simulink model "Excavator_Mevea_Bucket"  (R2026a)
settings: Solver=ode23t  StopTime=stopTime  FixedStep=1e-5  MaxStep=Ts  AbsTol=1e-3
PostLoadFcn:
  | set_param(bdroot,'IgnoredZcDiagnostic','none');
  | Excavator_Test_Scenario_Select('loadedBucketDigCycle');
  | Excavator_Mevea_params
StartFcn:
  | tStart = tic;
StopFcn:
  | elapsedSimTime = toc(tStart);
  | disp(['Elapsed Sim Time = ' num2str(elapsedSimTime)]);
model workspace: external: MAT-File ExcavatorAssemblyDataStruct.mat (data not in the file)
undefined symbols (not defined in the file or in its folder): AToBRegOrificeVector, AToTOrificeVector, BiPOrificeVector, BoomC, boomHEArea, boomREArea, boomUpMaxQ, boomValve, BToTOrificeVector, BucketC, bucketCloseMaxQ, bucketOpenMaxQ, BucketR, bucketValve, fluids, gravity, LeftBoomR, maxPumpDisp, minPumpDisp, nominalEngineSpeed, P28Assembly, PToAOrificeVector, PToBOrificeVector, pumpCmdNegRateLimit, pumpCmdPosRateLimit, RightBoomR, StickC, stickInMaxQ, stickOutMaxQ, StickR, stickValve, SwingC, swingDisplacement, swingHighSpeedThreshold, swingMaxQ, SwingR, swingSpeedQGain, swingValve, valveCmdNegRateLimit, valveCmdPosRateLimit, X, Y, Z
libraries: fl_lib x89, sm_lib x79, SimscapeFluids_lib x78, nesl_utility x57, simulink_extras x11, Excavator_Parts_Lib x6, SignalEditorBlockLib x1
(part 4 of 7)

== system Excavator_Mevea_Bucket/Excavator/Hydraulics/Functions/Bucket ==
  note: This leakage can be included if necessary.
      | Scale carefully to avoid drift due to gravity.
  BucketCylinder : SimscapeFluids_lib/Isothermal Liquid/Actuators/Double-Acting Actuator (IL)  single_fluid=true  mech_orientation=foundation.enum.MechOrientationTranslational.Positive  piston_area_A=bucketHEArea mm^2  piston_area_B=bucketREArea mm^2  stroke=bucketStroke mm  dead_volume_A=5e-4 m^3  dead_volume_B=5e-4 m^3  pressure_spec=foundation.enum.pressure_spec.atmospheric  environment_pressure=0.101325 MPa  hardstop_model=simscape.enum.hardstop.smooth  stiff_coeff=1e8 N/m  damping_coeff=1e6 N/(m/s)  transition=0.1 mm  coeff_rest=0.7  v_tol=0.001 m/s  f_tol=0.001 N  cushion_A_spec=simscape.enum.onoff.off  area_plunger_A=1e-4 m^2  length_plunger_A=1e-3 m  area_cushion_orifice_A=1e-6 m^2  area_leak_plunger_A=1e-7 m^2  p_crack_differential_A=0.01 MPa  press_max_differential_A=0.1 MPa  check_valve_area_max_A=1e-4 m^2  check_valve_area_leak_A=1e-10 m^2  smoothing_factor_A=0  cushion_B_spec=simscape.enum.onoff.off  area_plunger_B=1e-4 m^2  length_plunger_B=1e-3 m  area_cushion_orifice_B=1e-6 m^2  area_leak_plunger_B=1e-7 m^2  p_crack_differential_B=0.01 MPa  press_max_differential_B=0.1 MPa  check_valve_area_max_B=1e-4 m^2  check_valve_area_leak_B=1e-10 m^2  smoothing_factor_B=0  friction_spec=true  breakaway_Coulomb_ratio=bucketCylFriction.brkawyToCoulRatio  breakaway_velocity=bucketCylFriction.brkawyVel m/s  preload_force=bucketCylFriction.preloadForce N  Coulomb_coeff=bucketCylFriction.coulForceCoef N/Pa  viscous_coeff=bucketCylFriction.viscCoeff N/(m/s)  leakage_spec=simscape.enum.onoff.off  clearance=1e-4 m  piston_length=0.01 m  displacement_spec=foundation.enum.DisplacementSpec.Calculate  x0=initBucketPistonPos mm  dynamic_compressibility=simscape.enum.onoff.on  p0_A=initBucketHEPr bar  p0_B=initBucketREPr bar  p_nominal_A=0.101325 MPa  p_nominal_B=0.101325 MPa
  BucketHEPrSensor : fl_lib/Isothermal Liquid/Sensors/Pressure Sensor (IL)  pressure_measure=foundation.enum.pressure_measure.gauge
  BucketREPrSensor : fl_lib/Isothermal Liquid/Sensors/Pressure Sensor (IL)  pressure_measure=foundation.enum.pressure_measure.gauge
  BucketScope : Scope  NumInputPorts=3
      settings: ActiveDisplayYMinimum=-87.77863  ActiveDisplayYMaximum=1124.28313  DataLoggingVariableName=ScopeData2
  BucketTranslationalRef : fl_lib/Mechanical/Translational Elements/Mechanical Translational Reference
  Laminar Leakage (IL)1 : fl_lib/Isothermal Liquid/Elements/Laminar Leakage (IL)  Commented=on  cross_section_geometry=foundation.enum.cross_section_geometry.annular  diameter=1e-3 m  inner_diameter=bucketBoreDiameter-pistonCylClearance mm  outer_diameter=bucketBoreDiameter mm  width=1e-3 m  height=0.1 m  major_axis=1e-3 m  minor_axis=5e-4 m  side_length=1e-3 m  length=pistonHeadLen mm  resistance=1e3 MPa*s/m^3
  PS-Simulink Converter : nesl_utility/PS-Simulink Converter  PhysicalDomain=network_engine_domain  SubClassName=ps_output  LeftPortType=input  RightPortType=output  PseudoPeriodic=off  Frequencies=[]  VectorFormat=1-D array  Unit=bar  AffineConversion=off
  PS-Simulink Converter1 : nesl_utility/PS-Simulink Converter  PhysicalDomain=network_engine_domain  SubClassName=ps_output  LeftPortType=input  RightPortType=output  PseudoPeriodic=off  Frequencies=[]  VectorFormat=1-D array  Unit=bar  AffineConversion=off
  PS-Simulink Converter2 : nesl_utility/PS-Simulink Converter  PhysicalDomain=network_engine_domain  SubClassName=ps_output  LeftPortType=input  RightPortType=output  PseudoPeriodic=off  Frequencies=[]  VectorFormat=1-D array  Unit=mm  AffineConversion=off
  Simscape Bus : SimscapeBus  HierarchyStrings=BucketC;BucketR
  Transfer Fcn (with initial outputs) : simulink_extras/Additional Linear/Transfer Fcn (with initial outputs)  N=[1]  D="[0.01  1]"  Y0=initBucketHEPr  U0=initBucketHEPr
  Transfer Fcn (with initial outputs)1 : simulink_extras/Additional Linear/Transfer Fcn (with initial outputs)  N=[1]  D="[0.01  1]"  Y0=initBucketREPr  U0=initBucketREPr
  BucketA : PMIOPort  Side=Left
  BucketB : PMIOPort  Port=2  Side=Left
  BucketHydToMech : PMIOPort  Port=3  Side=Right
  BucketHEPr : Outport
  BucketREPr : Outport  Port=2
  BucketPos : Outport  Port=3
  wires:
  PS-Simulink Converter1/1 -> Transfer Fcn (with initial outputs)/1  "BucketHEPr"
  PS-Simulink Converter/1 -> Transfer Fcn (with initial outputs)1/1  "BucketREPr"
  Transfer Fcn (with initial outputs)/1 -> BucketScope/3, BucketHEPr/1  "BucketHEPr"
  Transfer Fcn (with initial outputs)1/1 -> BucketREPr/1, BucketScope/2  "BucketREPr"
  PS-Simulink Converter2/1 -> BucketScope/1, BucketPos/1  "BucketPos"
  connections:
  Simscape Bus/LConn2 -- BucketCylinder/RConn2
  BucketCylinder/LConn2 -- BucketA/RConn1 -- Laminar Leakage (IL)1/LConn1 -- BucketHEPrSensor/LConn1
  BucketCylinder/LConn1 -- Simscape Bus/LConn1 -- BucketTranslationalRef/LConn1
  BucketREPrSensor/LConn1 -- Laminar Leakage (IL)1/RConn1 -- BucketCylinder/RConn3 -- BucketB/RConn1
  Simscape Bus/RConn1 -- BucketHydToMech/RConn1
  BucketREPrSensor/RConn1 -- PS-Simulink Converter/LConn1
  BucketHEPrSensor/RConn1 -- PS-Simulink Converter1/LConn1
  PS-Simulink Converter2/LConn1 -- BucketCylinder/RConn1

== system Excavator_Mevea_Bucket/Excavator/Hydraulics/Functions/Stick ==
  note: This leakage can be included if necessary.
      | Scale carefully to avoid drift due to gravity.
  Laminar Leakage (IL)1 : fl_lib/Isothermal Liquid/Elements/Laminar Leakage (IL)  Commented=on  cross_section_geometry=foundation.enum.cross_section_geometry.annular  diameter=1e-3 m  inner_diameter=stickBoreDiameter-pistonCylClearance mm  outer_diameter=stickBoreDiameter mm  width=1e-3 m  height=0.1 m  major_axis=1e-3 m  minor_axis=5e-4 m  side_length=1e-3 m  length=pistonHeadLen mm  resistance=1e3 MPa*s/m^3
  PS-Simulink Converter : nesl_utility/PS-Simulink Converter  PhysicalDomain=network_engine_domain  SubClassName=ps_output  LeftPortType=input  RightPortType=output  PseudoPeriodic=off  Frequencies=[]  VectorFormat=1-D array  Unit=bar  AffineConversion=off
  PS-Simulink Converter1 : nesl_utility/PS-Simulink Converter  PhysicalDomain=network_engine_domain  SubClassName=ps_output  LeftPortType=input  RightPortType=output  PseudoPeriodic=off  Frequencies=[]  VectorFormat=1-D array  Unit=bar  AffineConversion=off
  PS-Simulink Converter2 : nesl_utility/PS-Simulink Converter  PhysicalDomain=network_engine_domain  SubClassName=ps_output  LeftPortType=input  RightPortType=output  PseudoPeriodic=off  Frequencies=[]  VectorFormat=1-D array  Unit=mm  AffineConversion=off
  Simscape Bus : SimscapeBus  HierarchyStrings=StickC;StickR
  StickCylinder : SimscapeFluids_lib/Isothermal Liquid/Actuators/Double-Acting Actuator (IL)  single_fluid=true  mech_orientation=foundation.enum.MechOrientationTranslational.Positive  piston_area_A=stickHEArea mm^2  piston_area_B=stickREArea mm^2  stroke=stickStroke mm  dead_volume_A=1e-3 m^3  dead_volume_B=1e-3 m^3  pressure_spec=foundation.enum.pressure_spec.atmospheric  environment_pressure=0.101325 MPa  hardstop_model=simscape.enum.hardstop.smooth  stiff_coeff=1e8 N/m  damping_coeff=1e5 N/(m/s)  transition=0.1 mm  coeff_rest=0.7  v_tol=0.001 m/s  f_tol=0.001 N  cushion_A_spec=simscape.enum.onoff.off  area_plunger_A=1e-4 m^2  length_plunger_A=1e-3 m  area_cushion_orifice_A=1e-6 m^2  area_leak_plunger_A=1e-7 m^2  p_crack_differential_A=0.01 MPa  press_max_differential_A=0.1 MPa  check_valve_area_max_A=1e-4 m^2  check_valve_area_leak_A=1e-10 m^2  smoothing_factor_A=0  cushion_B_spec=simscape.enum.onoff.off  area_plunger_B=1e-4 m^2  length_plunger_B=1e-3 m  area_cushion_orifice_B=1e-6 m^2  area_leak_plunger_B=1e-7 m^2  p_crack_differential_B=0.01 MPa  press_max_differential_B=0.1 MPa  check_valve_area_max_B=1e-4 m^2  check_valve_area_leak_B=1e-10 m^2  smoothing_factor_B=0  friction_spec=simscape.enum.onoff.on  breakaway_Coulomb_ratio=stickCylFriction.brkawyToCoulRatio  breakaway_velocity=stickCylFriction.brkawyVel m/s  preload_force=stickCylFriction.preloadForce N  Coulomb_coeff=stickCylFriction.coulForceCoef N/Pa  viscous_coeff=stickCylFriction.viscCoeff N/(m/s)  leakage_spec=simscape.enum.onoff.off  clearance=1e-4 m  piston_length=0.01 m  displacement_spec=foundation.enum.DisplacementSpec.Calculate  x0=initStickPistonPos mm  dynamic_compressibility=simscape.enum.onoff.on  p0_A=initStickHEPr bar  p0_B=initStickREPr bar  p_nominal_A=0.101325 MPa  p_nominal_B=0.101325 MPa
  StickHEPrSensor : fl_lib/Isothermal Liquid/Sensors/Pressure Sensor (IL)  pressure_measure=foundation.enum.pressure_measure.gauge
  StickREPrSensor : fl_lib/Isothermal Liquid/Sensors/Pressure Sensor (IL)  pressure_measure=foundation.enum.pressure_measure.gauge
  StickTranslationalRef : fl_lib/Mechanical/Translational Elements/Mechanical Translational Reference
  Transfer Fcn (with initial outputs) : simulink_extras/Additional Linear/Transfer Fcn (with initial outputs)  N=[1]  D="[0.01  1]"  Y0=initStickREPr  U0=initStickREPr
  Transfer Fcn (with initial outputs)1 : simulink_extras/Additional Linear/Transfer Fcn (with initial outputs)  N=[1]  D="[0.01  1]"  Y0=initStickHEPr  U0=initStickHEPr
  StickA : PMIOPort  Side=Left
  StickB : PMIOPort  Port=2  Side=Left
  StickHydToMech : PMIOPort  Port=3  Side=Right
  StickHEPr : Outport
  StickREPr : Outport  Port=2
  StickPos : Outport  Port=3
  wires:
  PS-Simulink Converter/1 -> Transfer Fcn (with initial outputs)/1  "StickREPr"
  PS-Simulink Converter1/1 -> Transfer Fcn (with initial outputs)1/1  "StickHEPr"
  Transfer Fcn (with initial outputs)/1 -> StickREPr/1  "StickREPr"
  PS-Simulink Converter2/1 -> StickPos/1  "StickPos"
  Transfer Fcn (with initial outputs)1/1 -> StickHEPr/1  "StickHEPr"
  connections:
  StickCylinder/RConn2 -- Simscape Bus/LConn2
  StickCylinder/RConn3 -- Laminar Leakage (IL)1/RConn1 -- StickREPrSensor/LConn1 -- StickB/RConn1
  StickHEPrSensor/LConn1 -- Laminar Leakage (IL)1/LConn1 -- StickCylinder/LConn2 -- StickA/RConn1
  StickTranslationalRef/LConn1 -- Simscape Bus/LConn1 -- StickCylinder/LConn1
  Simscape Bus/RConn1 -- StickHydToMech/RConn1
  StickREPrSensor/RConn1 -- PS-Simulink Converter/LConn1
  StickHEPrSensor/RConn1 -- PS-Simulink Converter1/LConn1
  PS-Simulink Converter2/LConn1 -- StickCylinder/RConn1

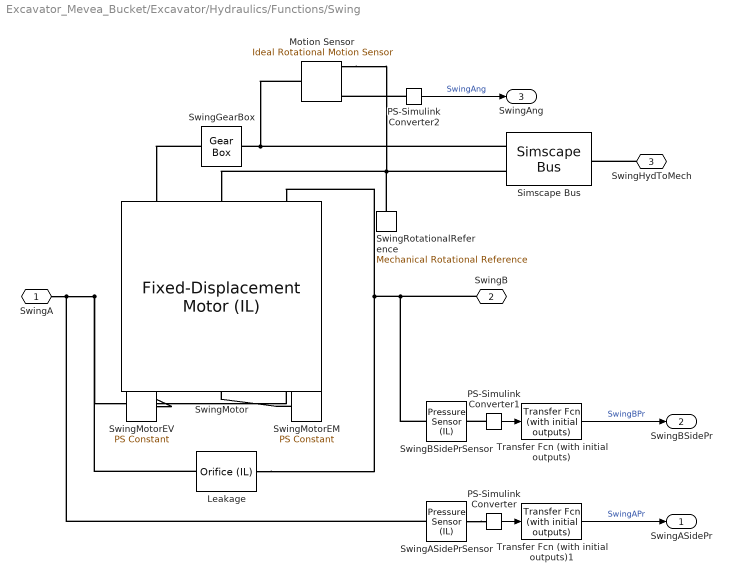
== system Excavator_Mevea_Bucket/Excavator/Hydraulics/Functions/Swing ==
  Leakage : SimscapeFluids_lib/Isothermal Liquid/Valves & Orifices/Orifices/Orifice (IL)  orifice_type=foundation.enum.constant_variable.constant  constant_orifice_spec=fluids.isothermal_liquid.valves_orifices.orifices.enum.constant_orifice_spec.area  variable_orifice_spec=fluids.isothermal_liquid.valves_orifices.orifices.enum.orifice_spec.linear  orifice_area_constant=5e-7 m^2  p_diff_TLU_constant=[-4, -3, -2, -1, -.5, 0, .5, 1, 2, 3, 4] MPa  vol_flow_TLU_constant=[-2.44, -2.12, -1.68, -1.22, -.84, 0, .85, 1.21, 1.7, 2.09, 2.41] .* 1e-3 m^3/s  S_min=0 m  del_S=5e-3 m  open_orientation=fluids.isothermal_liquid.valves_orifices.orifices.enum.orifice_orientation.positive  area_max=1e-4 m^2  area_leak=1e-10 m^2  S_TLU=[0, .002, .004, .007, .017] m  orifice_area_TLU=[1e-09, 2.0352e-07, 4.0736e-05, .00011438, .00034356] m^2  area=inf m^2  Cd=0.64  Re_c=150  smoothing_factor=0.01  pressure_recovery=false  S_vol_flow_TLU=[0, .002, .004, .007, .017] m  p_diff_TLU=[.3, .5, .7] MPa  vol_flow_TLU=1e-3 * [1.7e-05, 2e-05, 2.6e-05; .0035, .0045, .0053; .7, .9, 1.06; 1.96, 2.5, 3; 6, 7.7, 9.13] m^3/s
  Motion Sensor : fl_lib/Mechanical/Mechanical Sensors/Ideal Rotational Motion Sensor  reference=foundation.enum.MeasurementReference.difference  acceleration_port=false  velocity_port=true  position_port=true  wrap_angle=simscape.enum.onoff.off  offset=initSwingAngle deg
  PS-Simulink Converter : nesl_utility/PS-Simulink Converter  PhysicalDomain=network_engine_domain  SubClassName=ps_output  LeftPortType=input  RightPortType=output  PseudoPeriodic=off  Frequencies=[]  VectorFormat=1-D array  Unit=bar  AffineConversion=off
  PS-Simulink Converter1 : nesl_utility/PS-Simulink Converter  PhysicalDomain=network_engine_domain  SubClassName=ps_output  LeftPortType=input  RightPortType=output  PseudoPeriodic=off  Frequencies=[]  VectorFormat=1-D array  Unit=bar  AffineConversion=off
  PS-Simulink Converter2 : nesl_utility/PS-Simulink Converter  PhysicalDomain=network_engine_domain  SubClassName=ps_output  LeftPortType=input  RightPortType=output  PseudoPeriodic=off  Frequencies=[]  VectorFormat=1-D array  Unit=deg  AffineConversion=off
  Simscape Bus : SimscapeBus  HierarchyStrings=SwingR;SwingC
  SwingASidePrSensor : fl_lib/Isothermal Liquid/Sensors/Pressure Sensor (IL)  pressure_measure=foundation.enum.pressure_measure.gauge
  SwingBSidePrSensor : fl_lib/Isothermal Liquid/Sensors/Pressure Sensor (IL)  pressure_measure=foundation.enum.pressure_measure.gauge
  SwingGearBox : fl_lib/Mechanical/Mechanisms/Gear Box  ratio=swingGearRatio  t_in_specify=off  t_in_priority=None  t_in=0 N*m  t_in_nominal_specify=off  t_in_nominal_value=1  t_in_nominal_unit=N*m  t_out_specify=off  t_out_priority=None  t_out=0 N*m  t_out_nominal_specify=off  t_out_nominal_value=1  t_out_nominal_unit=N*m
  SwingMotor : SimscapeFluids_lib/Isothermal Liquid/Pumps & Motors/Fixed-Displacement Motor (IL)  leakage_friction_spec=fluids.isothermal_liquid.pumps_motors.enum.MotorLossSpec.InputEfficiency  displacement=swingDisplacement cm^3/rev  omega_nominal=188 rad/s  p_nominal=100e5 Pa  vol_eff_nominal=0.92  mech_eff_nominal=1 - (6283185.3072*(0.6e-6)/(swingDisplacement)) - (6283185.3072*(0.05)/(swingDisplacement)/(100e5))  no_load_torque=0.05 N*m  p_diff_eff_TLU=[100000, 1000000, 2000000] Pa  omega_eff_TLU=[25, 50, 100, 200, 300, 400] rad/s  vol_eff_TLU=[.816, .908, .954, .977, .981, .984; .325, .663, .831, .916, .925, .946; .137, .568, .78, .892, .893, .91]  mech_eff_TLU=[.996, .996, .996, .996, .996, .996; .988, .989, .989, .989, .989, .99; .981, .981, .982, .982, .983, .984]  p_diff_loss_TLU=[100000, 1000000, 2000000] Pa  omega_loss_TLU=[25, 50, 100, 200, 300, 400] rad/s  vol_loss_TLU=[.0282, .0253, .0241, .0235, .0291, .0325; .2596, .1271, .1017, .0917, .1216, .1142; .7874, .1901, .141, .1211, .1797, .1978] * 1e-3 m^3/s  mech_loss_TLU=[.002, .002, .002, .002, .002, .002; .06, .055, .055, .055, .055, .05; .19, .19, .18, .18, .17, .16] N*m  q_shaft_TLU=[.125, .25, .5, 1, 1.5, 2] * 1e-3 m^3/s  p_diff_shaft_TLU=[.1, 1, 2] MPa  torque_shaft_TLU=[.47, 4.72, 9.35; .47, 4.7, 9.36; .47, 4.7, 9.4; .47, 4.7, 9.41; .47, 4.7, 9.46; .47, 4.68, 9.5] N*m  omega_shaft_TLU=[205, 80, 35; 455, 330, 285; 955, 831, 780; 1950, 1830, 1780; 2940, 2775, 2680; 3940, 3780, 3640] rpm  vol_eff_min=1e-3  vol_eff_max=1  mech_eff_min=1e-3  mech_eff_max=1  pressure_threshold=1e5 Pa  omega_threshold=10 rad/s  supplied_range_check=simscape.enum.assert.action.none  motor_mode_check=simscape.enum.assert.action.none  pressure_check=simscape.enum.assert.action.none  p_min_valid=0 + 101325 Pa
  SwingMotorEM : fl_lib/Physical Signals/Sources/PS Constant  constant=1
  SwingMotorEV : fl_lib/Physical Signals/Sources/PS Constant  constant=1
  SwingRotationalReference : fl_lib/Mechanical/Rotational Elements/Mechanical Rotational Reference
  Transfer Fcn (with initial outputs) : simulink_extras/Additional Linear/Transfer Fcn (with initial outputs)  N=[1]  D="[0.01  1]"  Y0=initSwingBPr  U0=initSwingBPr
  Transfer Fcn (with initial outputs)1 : simulink_extras/Additional Linear/Transfer Fcn (with initial outputs)  N=[1]  D="[0.01  1]"  Y0=initSwingAPr  U0=initSwingAPr
  SwingA : PMIOPort  Side=Left
  SwingB : PMIOPort  Port=2  Side=Left
  SwingHydToMech : PMIOPort  Port=3  Side=Right
  SwingASidePr : Outport
  SwingBSidePr : Outport  Port=2
  SwingAng : Outport  Port=3
  wires:
  Transfer Fcn (with initial outputs)1/1 -> SwingASidePr/1  "SwingAPr"
  PS-Simulink Converter1/1 -> Transfer Fcn (with initial outputs)/1
  Transfer Fcn (with initial outputs)/1 -> SwingBSidePr/1  "SwingBPr"
  PS-Simulink Converter/1 -> Transfer Fcn (with initial outputs)1/1
  PS-Simulink Converter2/1 -> SwingAng/1  "SwingAng"
  connections:
  SwingGearBox/LConn1 -- SwingMotor/RConn1
  SwingMotorEM/RConn1 -- SwingMotor/LConn2
  SwingMotorEV/RConn1 -- SwingMotor/LConn1
  SwingHydToMech/RConn1 -- Simscape Bus/RConn1
  SwingRotationalReference/LConn1 -- Simscape Bus/LConn2 -- SwingMotor/RConn2 -- Motion Sensor/RConn1
  SwingASidePrSensor/RConn1 -- PS-Simulink Converter/LConn1
  PS-Simulink Converter1/LConn1 -- SwingBSidePrSensor/RConn1
  Simscape Bus/LConn1 -- Motion Sensor/LConn1 -- SwingGearBox/RConn1
  Leakage/RConn1 -- SwingMotor/RConn3 -- SwingBSidePrSensor/LConn1 -- SwingB/RConn1
  Leakage/LConn1 -- SwingASidePrSensor/LConn1 -- SwingA/RConn1 -- SwingMotor/LConn3
  PS-Simulink Converter2/LConn1 -- Motion Sensor/RConn3

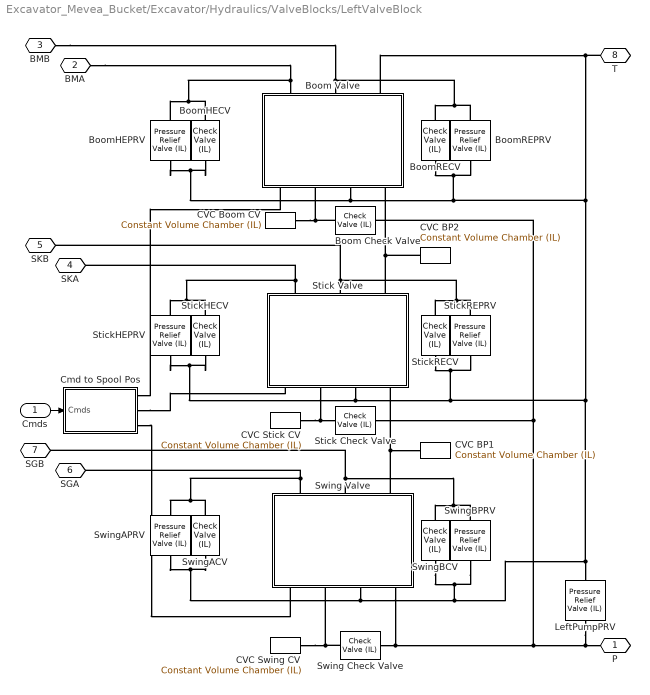
== system Excavator_Mevea_Bucket/Excavator/Hydraulics/ValveBlocks/LeftValveBlock ==
  Cmds : Inport
  Boom Check Valve : SimscapeFluids_lib/Isothermal Liquid/Valves & Orifices/Directional Control Valves/Check Valve (IL)  opening_spec=2*(fluids.isothermal_liquid.valves_orifices.enum.opening_spec.linear)-1  pressure_control_spec=fluids.isothermal_liquid.valves_orifices.enum.pressure_control_spec.dp  p_crack_differential=checkValves.crackingPrDiff bar  p_crack_gauge=0.1 MPa  press_max_differential=checkValves.maxOpeningPrDiff bar  press_max_gauge=0.2 MPa  area_max=checkValves.maxOpeningArea mm^2  area_leak="checkValves.leakageArea  mm^2"  p_diff_TLU=[0.01 : 0.01 : 0.1] MPa  valve_area_TLU=[1e-10, 1e-05, 2e-05, 3e-05, 4e-05, 5e-05, 6e-05, 7.5e-05, 8.5e-05, .0001] m^2  vol_flow_TLU=[.000358, .045, .11, .191, .284, .39, .505, .63, .764, .905] .* 1e-3 m^3/s  area=inf m^2  Cd=0.7  Re_c=150  smoothing_factor=0.1  pressure_recovery=simscape.enum.onoff.off  opening_dynamics=simscape.enum.onoff.off  tau=0.1 s
  Boom Valve : Subsystem  mask{valveData=boomValve}
      mask prompts: valveData "Boom Valve Data Structure:"
      mask DialogControl DescGroupVar Prompt: Boom Valve
      mask DialogControl DescTextVar Prompt: The Boom Valve is a 6/3 valve with integrated check valve for induced flow.
      mask Display: image('Valve_6p3w_chkVAT_IMAGE.png');
  BoomHECV : SimscapeFluids_lib/Isothermal Liquid/Valves & Orifices/Directional Control Valves/Check Valve (IL)  opening_spec=2*(fluids.isothermal_liquid.valves_orifices.enum.opening_spec.linear)-1  pressure_control_spec=fluids.isothermal_liquid.valves_orifices.enum.pressure_control_spec.dp  p_crack_differential=checkValves.crackingPrDiff bar  p_crack_gauge=0.1 MPa  press_max_differential=checkValves.maxOpeningPrDiff bar  press_max_gauge=0.2 MPa  area_max=checkValves.maxOpeningArea mm^2  area_leak=checkValves.leakageArea mm^2  p_diff_TLU=[0.01 : 0.01 : 0.1] MPa  valve_area_TLU=[1e-10, 1e-05, 2e-05, 3e-05, 4e-05, 5e-05, 6e-05, 7.5e-05, 8.5e-05, .0001] m^2  vol_flow_TLU=[.000358, .045, .11, .191, .284, .39, .505, .63, .764, .905] .* 1e-3 m^3/s  area=inf m^2  Cd=0.64  Re_c=150  smoothing_factor=0.01  pressure_recovery=simscape.enum.onoff.off  opening_dynamics=simscape.enum.onoff.off  tau=0.1 s
  BoomHEPRV : SimscapeFluids_lib/Isothermal Liquid/Valves & Orifices/Pressure Control Valves/Pressure Relief Valve (IL)  set_pressure_spec=foundation.enum.constant_controlled.constant  opening_spec=fluids.isothermal_liquid.valves_orifices.enum.opening_spec.linear  pressure_spec=fluids.isothermal_liquid.valves_orifices.enum.pressure_control_spec.dp  p_set_gauge=0.1 MPa  p_set_differential=fcnPRV.reliefPr bar  p_range=fcnPRV.regRange bar  area_max=fcnPRV.maxOpeningArea mm^2  area_leak=fcnPRV.leakageArea mm^2  p_diff_TLU=[0.2 : 0.2 : 1.2] MPa  p_gauge_TLU=[0.2 : 0.2 : 1.2] MPa  valve_area_TLU=[1e-10, 2e-06, 4e-06, 6e-06, 8e-06, 1e-05] m^2  vol_flow_TLU=[1e-09, 3.6e-05, 8.9e-05, .00015, .00023, .00031] m^3/s  area=inf m^2  Cd=0.64  Re_c=150  smoothing_factor=0.01  pressure_recovery=simscape.enum.onoff.off  opening_dynamics=simscape.enum.onoff.off  tau=0.1 s
  BoomRECV : SimscapeFluids_lib/Isothermal Liquid/Valves & Orifices/Directional Control Valves/Check Valve (IL)  opening_spec=2*(fluids.isothermal_liquid.valves_orifices.enum.opening_spec.linear)-1  pressure_control_spec=fluids.isothermal_liquid.valves_orifices.enum.pressure_control_spec.dp  p_crack_differential=checkValves.crackingPrDiff bar  p_crack_gauge=0.1 MPa  press_max_differential=checkValves.maxOpeningPrDiff bar  press_max_gauge=0.2 MPa  area_max=checkValves.maxOpeningArea mm^2  area_leak=checkValves.leakageArea mm^2  p_diff_TLU=[0.01 : 0.01 : 0.1] MPa  valve_area_TLU=[1e-10, 1e-05, 2e-05, 3e-05, 4e-05, 5e-05, 6e-05, 7.5e-05, 8.5e-05, .0001] m^2  vol_flow_TLU=[.000358, .045, .11, .191, .284, .39, .505, .63, .764, .905] .* 1e-3 m^3/s  area=inf m^2  Cd=0.64  Re_c=150  smoothing_factor=0.01  pressure_recovery=simscape.enum.onoff.off  opening_dynamics=simscape.enum.onoff.off  tau=0.1 s
  BoomREPRV : SimscapeFluids_lib/Isothermal Liquid/Valves & Orifices/Pressure Control Valves/Pressure Relief Valve (IL)  set_pressure_spec=foundation.enum.constant_controlled.constant  opening_spec=fluids.isothermal_liquid.valves_orifices.enum.opening_spec.linear  pressure_spec=fluids.isothermal_liquid.valves_orifices.enum.pressure_control_spec.dp  p_set_gauge=0.1 MPa  p_set_differential=fcnPRV.reliefPr bar  p_range=fcnPRV.regRange bar  area_max=fcnPRV.maxOpeningArea mm^2  area_leak=fcnPRV.leakageArea mm^2  p_diff_TLU=[0.2 : 0.2 : 1.2] MPa  p_gauge_TLU=[0.2 : 0.2 : 1.2] MPa  valve_area_TLU=[1e-10, 2e-06, 4e-06, 6e-06, 8e-06, 1e-05] m^2  vol_flow_TLU=[1e-09, 3.6e-05, 8.9e-05, .00015, .00023, .00031] m^3/s  area=inf m^2  Cd=0.64  Re_c=150  smoothing_factor=0.01  pressure_recovery=simscape.enum.onoff.off  opening_dynamics=simscape.enum.onoff.off  tau=0.1 s
  CVC BP1 : fl_lib/Isothermal Liquid/Elements/Constant Volume Chamber (IL)  volume=vcVol m^3  p_I_specify=on  p_I_priority=High  p_I=p0 bar  p_I_nominal_specify=off  p_I_nominal_value=1  p_I_nominal_unit=MPa
  CVC BP2 : fl_lib/Isothermal Liquid/Elements/Constant Volume Chamber (IL)  volume=vcVol m^3  p_I_specify=on  p_I_priority=High  p_I=p0 bar  p_I_nominal_specify=off  p_I_nominal_value=1  p_I_nominal_unit=MPa
  CVC Boom CV : fl_lib/Isothermal Liquid/Elements/Constant Volume Chamber (IL)  volume=vcVol m^3  p_I_specify=on  p_I_priority=High  p_I=p0 bar  p_I_nominal_specify=off  p_I_nominal_value=1  p_I_nominal_unit=MPa
  CVC Stick CV : fl_lib/Isothermal Liquid/Elements/Constant Volume Chamber (IL)  volume=vcVol m^3  p_I_specify=on  p_I_priority=High  p_I=p0 bar  p_I_nominal_specify=off  p_I_nominal_value=1  p_I_nominal_unit=MPa
  CVC Swing CV : fl_lib/Isothermal Liquid/Elements/Constant Volume Chamber (IL)  volume=vcVol m^3  p_I_specify=on  p_I_priority=High  p_I=p0 bar  p_I_nominal_specify=off  p_I_nominal_value=1  p_I_nominal_unit=MPa
  Cmd to Spool Pos : Subsystem
  LeftPumpPRV : SimscapeFluids_lib/Isothermal Liquid/Valves & Orifices/Pressure Control Valves/Pressure Relief Valve (IL)  set_pressure_spec=foundation.enum.constant_controlled.constant  opening_spec=fluids.isothermal_liquid.valves_orifices.enum.opening_spec.linear  pressure_spec=fluids.isothermal_liquid.valves_orifices.enum.pressure_control_spec.dp  p_set_gauge=0.1 MPa  p_set_differential=pumpPRV.reliefPr bar  p_range=pumpPRV.regRange bar  area_max=pumpPRV.maxOpeningArea mm^2  area_leak=pumpPRV.leakageArea mm^2  p_diff_TLU=[30.15e5 : 15e3 : 31.35e5] Pa  p_gauge_TLU=[30.15e5 : 15e3 : 31.35e5] Pa  valve_area_TLU=[1 : 1 : 9] .* 1e-5 m^2  vol_flow_TLU=[1e-09, 3.6e-05, 8.9e-05, .00015, .00023, .00031] m^3/s  area=inf m^2  Cd=0.64  Re_c=150  smoothing_factor=0.1  pressure_recovery=simscape.enum.onoff.off  opening_dynamics=simscape.enum.onoff.off  tau=0.1 s
  Stick Check Valve : SimscapeFluids_lib/Isothermal Liquid/Valves & Orifices/Directional Control Valves/Check Valve (IL)  opening_spec=2*(fluids.isothermal_liquid.valves_orifices.enum.opening_spec.linear)-1  pressure_control_spec=fluids.isothermal_liquid.valves_orifices.enum.pressure_control_spec.dp  p_crack_differential=checkValves.crackingPrDiff bar  p_crack_gauge=0.1 MPa  press_max_differential=checkValves.maxOpeningPrDiff bar  press_max_gauge=0.2 MPa  area_max=checkValves.maxOpeningArea mm^2  area_leak="checkValves.leakageArea  mm^2"  p_diff_TLU=[0.01 : 0.01 : 0.1] MPa  valve_area_TLU=[1e-10, 1e-05, 2e-05, 3e-05, 4e-05, 5e-05, 6e-05, 7.5e-05, 8.5e-05, .0001] m^2  vol_flow_TLU=[.000358, .045, .11, .191, .284, .39, .505, .63, .764, .905] .* 1e-3 m^3/s  area=inf m^2  Cd=0.7  Re_c=150  smoothing_factor=0.1  pressure_recovery=simscape.enum.onoff.off  opening_dynamics=simscape.enum.onoff.off  tau=0.1 s
  Stick Valve : Subsystem  mask{valveData=stickValve}
      mask prompts: valveData "Stick Valve Data Structure:"
      mask DialogControl DescGroupVar Prompt: Stick Valve
      mask DialogControl DescTextVar Prompt: The Stick Valve is a 6/3 valve with integrated check valve for induced flow.
      mask Display: image('Valve_6p3w_chkVPA_IMAGE.png');
  StickHECV : SimscapeFluids_lib/Isothermal Liquid/Valves & Orifices/Directional Control Valves/Check Valve (IL)  opening_spec=2*(fluids.isothermal_liquid.valves_orifices.enum.opening_spec.linear)-1  pressure_control_spec=fluids.isothermal_liquid.valves_orifices.enum.pressure_control_spec.dp  p_crack_differential=checkValves.crackingPrDiff bar  p_crack_gauge=0.1 MPa  press_max_differential=checkValves.maxOpeningPrDiff bar  press_max_gauge=0.2 MPa  area_max=checkValves.maxOpeningArea mm^2  area_leak=checkValves.leakageArea mm^2  p_diff_TLU=[0.01 : 0.01 : 0.1] MPa  valve_area_TLU=[1e-10, 1e-05, 2e-05, 3e-05, 4e-05, 5e-05, 6e-05, 7.5e-05, 8.5e-05, .0001] m^2  vol_flow_TLU=[.000358, .045, .11, .191, .284, .39, .505, .63, .764, .905] .* 1e-3 m^3/s  area=inf m^2  Cd=0.64  Re_c=150  smoothing_factor=0.01  pressure_recovery=simscape.enum.onoff.off  opening_dynamics=simscape.enum.onoff.off  tau=0.1 s
  StickHEPRV : SimscapeFluids_lib/Isothermal Liquid/Valves & Orifices/Pressure Control Valves/Pressure Relief Valve (IL)  set_pressure_spec=foundation.enum.constant_controlled.constant  opening_spec=fluids.isothermal_liquid.valves_orifices.enum.opening_spec.linear  pressure_spec=fluids.isothermal_liquid.valves_orifices.enum.pressure_control_spec.dp  p_set_gauge=0.1 MPa  p_set_differential=fcnPRV.reliefPr bar  p_range=fcnPRV.regRange bar  area_max=fcnPRV.maxOpeningArea mm^2  area_leak=fcnPRV.leakageArea mm^2  p_diff_TLU=[0.2 : 0.2 : 1.2] MPa  p_gauge_TLU=[0.2 : 0.2 : 1.2] MPa  valve_area_TLU=[1e-10, 2e-06, 4e-06, 6e-06, 8e-06, 1e-05] m^2  vol_flow_TLU=[1e-09, 3.6e-05, 8.9e-05, .00015, .00023, .00031] m^3/s  area=inf m^2  Cd=0.64  Re_c=150  smoothing_factor=0.01  pressure_recovery=simscape.enum.onoff.off  opening_dynamics=simscape.enum.onoff.off  tau=0.1 s
  StickRECV : SimscapeFluids_lib/Isothermal Liquid/Valves & Orifices/Directional Control Valves/Check Valve (IL)  opening_spec=2*(fluids.isothermal_liquid.valves_orifices.enum.opening_spec.linear)-1  pressure_control_spec=fluids.isothermal_liquid.valves_orifices.enum.pressure_control_spec.dp  p_crack_differential=checkValves.crackingPrDiff bar  p_crack_gauge=0.1 MPa  press_max_differential=checkValves.maxOpeningPrDiff bar  press_max_gauge=0.2 MPa  area_max=checkValves.maxOpeningArea mm^2  area_leak=checkValves.leakageArea mm^2  p_diff_TLU=[0.01 : 0.01 : 0.1] MPa  valve_area_TLU=[1e-10, 1e-05, 2e-05, 3e-05, 4e-05, 5e-05, 6e-05, 7.5e-05, 8.5e-05, .0001] m^2  vol_flow_TLU=[.000358, .045, .11, .191, .284, .39, .505, .63, .764, .905] .* 1e-3 m^3/s  area=inf m^2  Cd=0.64  Re_c=150  smoothing_factor=0.01  pressure_recovery=simscape.enum.onoff.off  opening_dynamics=simscape.enum.onoff.off  tau=0.1 s
  StickREPRV : SimscapeFluids_lib/Isothermal Liquid/Valves & Orifices/Pressure Control Valves/Pressure Relief Valve (IL)  set_pressure_spec=foundation.enum.constant_controlled.constant  opening_spec=fluids.isothermal_liquid.valves_orifices.enum.opening_spec.linear  pressure_spec=fluids.isothermal_liquid.valves_orifices.enum.pressure_control_spec.dp  p_set_gauge=0.1 MPa  p_set_differential=fcnPRV.reliefPr bar  p_range=fcnPRV.regRange bar  area_max=fcnPRV.maxOpeningArea mm^2  area_leak=fcnPRV.leakageArea mm^2  p_diff_TLU=[0.2 : 0.2 : 1.2] MPa  p_gauge_TLU=[0.2 : 0.2 : 1.2] MPa  valve_area_TLU=[1e-10, 2e-06, 4e-06, 6e-06, 8e-06, 1e-05] m^2  vol_flow_TLU=[1e-09, 3.6e-05, 8.9e-05, .00015, .00023, .00031] m^3/s  area=inf m^2  Cd=0.64  Re_c=150  smoothing_factor=0.01  pressure_recovery=simscape.enum.onoff.off  opening_dynamics=simscape.enum.onoff.off  tau=0.1 s
  Swing Check Valve : SimscapeFluids_lib/Isothermal Liquid/Valves & Orifices/Directional Control Valves/Check Valve (IL)  opening_spec=2*(fluids.isothermal_liquid.valves_orifices.enum.opening_spec.linear)-1  pressure_control_spec=fluids.isothermal_liquid.valves_orifices.enum.pressure_control_spec.dp  p_crack_differential=checkValves.crackingPrDiff bar  p_crack_gauge=0.1 MPa  press_max_differential=checkValves.maxOpeningPrDiff bar  press_max_gauge=0.2 MPa  area_max=checkValves.maxOpeningArea mm^2  area_leak="checkValves.leakageArea  mm^2"  p_diff_TLU=[0.01 : 0.01 : 0.1] MPa  valve_area_TLU=[1e-10, 1e-05, 2e-05, 3e-05, 4e-05, 5e-05, 6e-05, 7.5e-05, 8.5e-05, .0001] m^2  vol_flow_TLU=[.000358, .045, .11, .191, .284, .39, .505, .63, .764, .905] .* 1e-3 m^3/s  area=inf m^2  Cd=0.7  Re_c=150  smoothing_factor=0.1  pressure_recovery=simscape.enum.onoff.off  opening_dynamics=simscape.enum.onoff.off  tau=0.1 s
  Swing Valve : Subsystem  mask{valveData=swingValve}
      mask prompts: valveData "Swing Valve Data Structure:"
      mask DialogControl DescGroupVar Prompt: Swing Valve
      mask DialogControl DescTextVar Prompt: The Swing Valve is a 6/3 valve.
      mask Display: image('Valve_6p3w_IMAGE.png');
  SwingACV : SimscapeFluids_lib/Isothermal Liquid/Valves & Orifices/Directional Control Valves/Check Valve (IL)  opening_spec=2*(fluids.isothermal_liquid.valves_orifices.enum.opening_spec.linear)-1  pressure_control_spec=fluids.isothermal_liquid.valves_orifices.enum.pressure_control_spec.dp  p_crack_differential=checkValves.crackingPrDiff bar  p_crack_gauge=0.1 MPa  press_max_differential=checkValves.maxOpeningPrDiff bar  press_max_gauge=0.2 MPa  area_max=checkValves.maxOpeningArea mm^2  area_leak=checkValves.leakageArea mm^2  p_diff_TLU=[0.01 : 0.01 : 0.1] MPa  valve_area_TLU=[1e-10, 1e-05, 2e-05, 3e-05, 4e-05, 5e-05, 6e-05, 7.5e-05, 8.5e-05, .0001] m^2  vol_flow_TLU=[.000358, .045, .11, .191, .284, .39, .505, .63, .764, .905] .* 1e-3 m^3/s  area=inf m^2  Cd=0.64  Re_c=150  smoothing_factor=0.01  pressure_recovery=simscape.enum.onoff.off  opening_dynamics=simscape.enum.onoff.off  tau=0.1 s
  SwingAPRV : SimscapeFluids_lib/Isothermal Liquid/Valves & Orifices/Pressure Control Valves/Pressure Relief Valve (IL)  set_pressure_spec=foundation.enum.constant_controlled.constant  opening_spec=fluids.isothermal_liquid.valves_orifices.enum.opening_spec.linear  pressure_spec=fluids.isothermal_liquid.valves_orifices.enum.pressure_control_spec.dp  p_set_gauge=0.1 MPa  p_set_differential=swingPRV.reliefPr bar  p_range=swingPRV.regRange bar  area_max=swingPRV.maxOpeningArea mm^2  area_leak=swingPRV.leakageArea mm^2  p_diff_TLU=[0.2 : 0.2 : 1.2] MPa  p_gauge_TLU=[0.2 : 0.2 : 1.2] MPa  valve_area_TLU=[1e-10, 2e-06, 4e-06, 6e-06, 8e-06, 1e-05] m^2  vol_flow_TLU=[1e-09, 3.6e-05, 8.9e-05, .00015, .00023, .00031] m^3/s  area=inf m^2  Cd=0.64  Re_c=150  smoothing_factor=0.01*5  pressure_recovery=simscape.enum.onoff.off  opening_dynamics=false  tau=0.1 s
  SwingBCV : SimscapeFluids_lib/Isothermal Liquid/Valves & Orifices/Directional Control Valves/Check Valve (IL)  opening_spec=2*(fluids.isothermal_liquid.valves_orifices.enum.opening_spec.linear)-1  pressure_control_spec=fluids.isothermal_liquid.valves_orifices.enum.pressure_control_spec.dp  p_crack_differential=checkValves.crackingPrDiff bar  p_crack_gauge=0.1 MPa  press_max_differential=checkValves.maxOpeningPrDiff bar  press_max_gauge=0.2 MPa  area_max=checkValves.maxOpeningArea mm^2  area_leak=checkValves.leakageArea mm^2  p_diff_TLU=[0.01 : 0.01 : 0.1] MPa  valve_area_TLU=[1e-10, 1e-05, 2e-05, 3e-05, 4e-05, 5e-05, 6e-05, 7.5e-05, 8.5e-05, .0001] m^2  vol_flow_TLU=[.000358, .045, .11, .191, .284, .39, .505, .63, .764, .905] .* 1e-3 m^3/s  area=inf m^2  Cd=0.64  Re_c=150  smoothing_factor=0.01  pressure_recovery=simscape.enum.onoff.off  opening_dynamics=simscape.enum.onoff.off  tau=0.1 s
  SwingBPRV : SimscapeFluids_lib/Isothermal Liquid/Valves & Orifices/Pressure Control Valves/Pressure Relief Valve (IL)  set_pressure_spec=foundation.enum.constant_controlled.constant  opening_spec=fluids.isothermal_liquid.valves_orifices.enum.opening_spec.linear  pressure_spec=fluids.isothermal_liquid.valves_orifices.enum.pressure_control_spec.dp  p_set_gauge=0.1 MPa  p_set_differential=swingPRV.reliefPr bar  p_range=swingPRV.regRange bar  area_max=swingPRV.maxOpeningArea mm^2  area_leak=swingPRV.leakageArea mm^2  p_diff_TLU=[0.2 : 0.2 : 1.2] MPa  p_gauge_TLU=[0.2 : 0.2 : 1.2] MPa  valve_area_TLU=[1e-10, 2e-06, 4e-06, 6e-06, 8e-06, 1e-05] m^2  vol_flow_TLU=[1e-09, 3.6e-05, 8.9e-05, .00015, .00023, .00031] m^3/s  area=inf m^2  Cd=0.64  Re_c=150  smoothing_factor=0.01*5  pressure_recovery=simscape.enum.onoff.off  opening_dynamics=false  tau=0.1 s
  P : PMIOPort  Side=Left
  BMA : PMIOPort  Port=2  Side=Right
  BMB : PMIOPort  Port=3  Side=Right
  SKA : PMIOPort  Port=4  Side=Right
  SKB : PMIOPort  Port=5  Side=Right
  SGA : PMIOPort  Port=6  Side=Right
  SGB : PMIOPort  Port=7  Side=Right
  T : PMIOPort  Port=8  Side=Right
  wires:
  Cmds/1 -> Cmd to Spool Pos/1(Cmds)
  connections:
  Swing Check Valve/LConn1 -- Swing Valve/LConn4 -- LeftPumpPRV/LConn1 -- P/RConn1 -- Stick Check Valve/LConn1 -- Boom Check Valve/LConn1
  StickHEPRV/LConn1 -- StickHECV/RConn1 -- SKA/RConn1 -- Stick Valve/RConn1
  SGB/RConn1 -- SwingBPRV/LConn1 -- SwingBCV/RConn1 -- Swing Valve/RConn2
  Boom Valve/LConn3 -- T/RConn1 -- Boom Valve/RConn3 -- LeftPumpPRV/RConn1 -- SwingBPRV/RConn1 -- SwingBCV/LConn1 -- SwingACV/LConn1 -- SwingAPRV/RConn1 -- Swing Valve/LConn3 -- StickHECV/LConn1 -- StickHEPRV/RConn1 -- Stick Valve/LConn3 -- StickREPRV/RConn1 -- StickRECV/LConn1 -- BoomREPRV/RConn1 -- BoomRECV/LConn1 -- BoomHECV/LConn1 -- BoomHEPRV/RConn1
  BoomHECV/RConn1 -- BMA/RConn1 -- Boom Valve/RConn1 -- BoomHEPRV/LConn1
  SwingACV/RConn1 -- Swing Valve/RConn1 -- SGA/RConn1 -- SwingAPRV/LConn1
  Boom Valve/RConn2 -- BoomREPRV/LConn1 -- BoomRECV/RConn1 -- BMB/RConn1
  Stick Valve/RConn2 -- StickREPRV/LConn1 -- StickRECV/RConn1 -- SKB/RConn1
  Swing Valve/RConn3 -- Stick Valve/LConn4 -- CVC BP1/LConn1
  Stick Valve/LConn2 -- CVC Stick CV/LConn1 -- Stick Check Valve/RConn1
  Stick Valve/RConn3 -- CVC BP2/LConn1 -- Boom Valve/LConn4
  Swing Check Valve/RConn1 -- CVC Swing CV/LConn1 -- Swing Valve/LConn2
  Cmd to Spool Pos/RConn3 -- Swing Valve/LConn1
  Boom Check Valve/RConn1 -- CVC Boom CV/LConn1 -- Boom Valve/LConn2
  Cmd to Spool Pos/RConn2 -- Stick Valve/LConn1
  Cmd to Spool Pos/RConn1 -- Boom Valve/LConn1
